simulink model "zad335a_Sim"  (Simulink 7.1)
settings: Solver=ode45  StartTime=0.0  StopTime=15.0  RelTol=1e-3
settings Model: Creator=mestar  LastModifiedBy=mestar

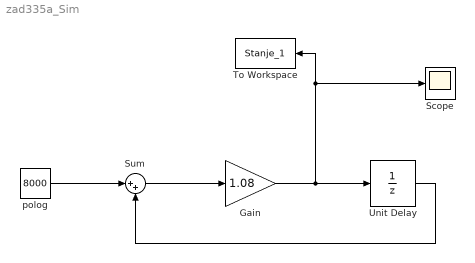
== system zad335a_Sim ==
  Gain : Gain  Gain=1.08  ParameterDataType=sfix(16)  ParameterScaling=2^0  OutDataType=sfix(16)  OutScaling=2^0
  Scope : Scope
  Sum : Sum  Inputs=|++  OutDataType=sfix(16)  OutScaling=2^0
  To Workspace : ToWorkspace  VariableName=Stanje_1  SampleTime=-1  SaveFormat=Array
  Unit Delay : UnitDelay
  polog : Constant  Value=8000  OutDataType=sfix(16)  OutScaling=2^0
  wires:
  polog/1 -> Sum/1
  Sum/1 -> Gain/1
  Gain/1 -> Unit Delay/1, To Workspace/1, Scope/1
  Unit Delay/1 -> Sum/2
